simulink model "sim"  (R2017a)
settings: Solver=VariableStepAuto  StartTime=0.0  StopTime=10.0  RelTol=1e-3
settings Model: Creator=Piotr Chudalewski  LastModifiedBy=Piotr Chudalewski

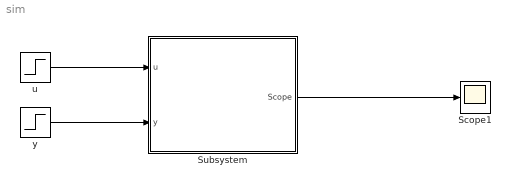
== system sim ==
  Scope1 : Scope
  Subsystem : Subsystem  mask{A=[ 1 1; 0 1], B=[2;3], C=[1 3], L=[-13;6]}
      mask prompts: A "Matrix A"; B "Matrix B"; C "Matrix C"; L "Matrix L"
      mask init:
      | x0 = eye(size(A,1))
      | x0_d = zeros(size(A,1),size(A,1)+1)
      | x0_d(1:size(A,1),1:size(A,1)) = x0;
      | x0_d
      | x0_vec=reshape(x0_d,[],1)
      | x0=x0_vec
      | 
      | 
      | %A = [1 2; 3 4];
      | s = (size(A,1)+1)*size(A);
      | A_d = zeros(s);
      | n = size(A,1);
      | 
      | for count = 1:n+1
      |     n_s = (count-1)*n+1;
      |     n_e = n_s+n-1;
      |     A_d(n_s:n_e,n_s:n_e) = A;
      | end
      | A=A_d
      | 
      | %B = [2;3];
      | s = (size(B,1)+1)*size(B);
      | B_d = zeros(s);
      | n_r = size(B_d,1);
      | n_c = size(B_d,2);
      | n_r_B = size(B,1)
      | n_c_B = size(B,2)
      | c=1;
      | for r = 1:n_r_B:n_r
      |     
      |     %for c = 1:n_c_B:n_c
      |         B_d(r:(n_r_B+r-1),c:n_c_B+c-1) = B;
      |         c=c+n_c_B;
      |        
      |     %end
      | end
      | B=B_d
      | 
      | %C = [11 3];
      | s = (size(C,1))*(1+size(C,2));
      | C_d = zeros(s);
      | n_r = size(C_d,1);
      | n_c = size(C_d,2);
      | n_r_C = size(C,1)
      | n_c_C = size(C,2)
      | c=1;
      | for r = 1:n_r_C:n_r
      |     
      |     %for c = 1:n_c_B:n_c
      |         C_d(r:(n_r_C+r-1),c:n_c_C+c-1) = C;
      |         c=c+n_c_C;
      |        
      |     %end
      | end
      | C=C_d
      | 
      | %L = [-2;3];
      | s = (size(L,1)+1)*size(L);
      | L_d = zeros(s);
      | n_r = size(L_d,1);
      | n_c = size(L_d,2);
      | n_r_L = size(L,1)
      | n_c_L = size(L,2)
      | c=1;
      | for r = 1:n_r_L:n_r
      |     
      |     %for c = 1:n_c_B:n_c
      |         L_d(r:(n_r_L+r-1),c:n_c_L+c-1) = L;
      |         c=c+n_c_L;
      |        
      |     %end
      | end
      | L=L_d
  u : Step  Before=[0 ;0; 0]  SampleTime=0
  y : Step  Before=[0;0;0]  SampleTime=0
  wires:
  u/1 -> Subsystem/1(u)
  Subsystem/1(Scope) -> Scope1/1
  y/1 -> Subsystem/2(y)

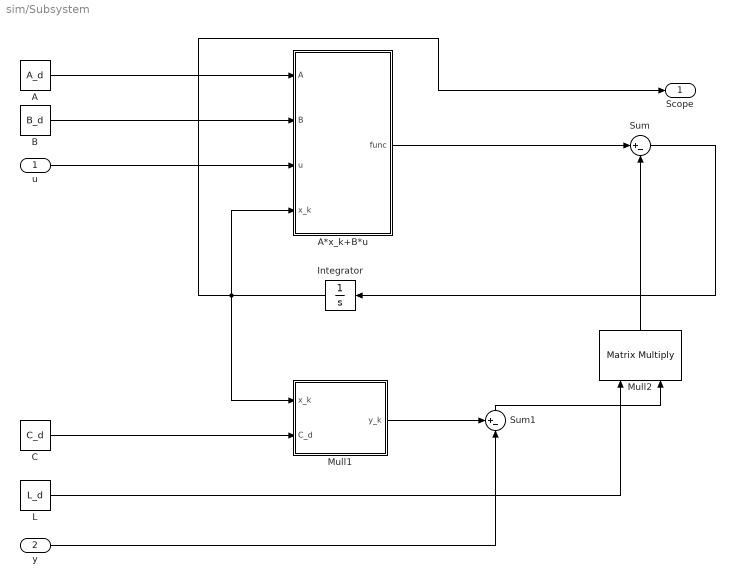
== system sim/Subsystem ==
  u : Inport
  y : Inport  Port=2
  A : Constant  Value=A_d
  "A*x_k+B*u " : MATLAB Function  TreatAsAtomicUnit=on
  "B " : Constant  Value=B_d
  "C " : Constant  Value=C_d  VectorParams1D=off
  Integrator : Integrator  InitialCondition=x0
  L : Constant  Value=L_d
  Mull1 : MATLAB Function  TreatAsAtomicUnit=on
  Mull2 : Product  Multiplication=Matrix(*)
  Sum : Sum  Inputs=|+-
  Sum1 : Sum  Inputs=+-|
  Scope : Outport
  wires:
  Mull2/1 -> Sum/2
  Sum/1 -> Integrator/1
  A/1 -> "A*x_k+B*u "/1(A)
  Sum1/1 -> Mull2/2
  "A*x_k+B*u "/1(func) -> Sum/1
  Integrator/1 -> Mull1/1(x_k), "A*x_k+B*u "/4(x_k), Scope/1
  u/1 -> "A*x_k+B*u "/3(u)
  "C "/1 -> Mull1/2(C_d)
  y/1 -> Sum1/2
  L/1 -> Mull2/1
  "B "/1 -> "A*x_k+B*u "/2(B)
  Mull1/1(y_k) -> Sum1/1

== matlab function sim/Subsystem/A*x_k+B*u  ==
  data: A input; B input; u input; x_k input; func output
function func = fcn(A, B, u, x_k)
% n -> stan
% p -> wyjście
% m -> wejście
%A -> R(n * n)
%B -> R(n * m)
%A : 2x2


%testowe A i B
%A = [1 0; 0 1];
%B = [1 0 0;0 1 1];



func = A*x_k+B*u;

== matlab function sim/Subsystem/Mull1 ==
  data: x_k input; C_d input; y_k output
function y_k = fcn(x_k,C_d)
% n -> stan
% p -> wyjście
% m -> wejście
%A -> R(n * n)
%B -> R(n * m)
%A : 2x2


%testowe A i B
%A = [1 0; 0 1];
%B = [1 0 0;0 1 1];



y_k = C_d*x_k;
